simulink model "sf_tlevery"  (Simulink 6.0)
settings: Solver=ode45  StartTime=0.0  StopTime=100  RelTol=1e-3
settings Model: CovMetricSettings=dcmtr  Creator=The MathWorks Inc.  LastModifiedBy=batserve  ExtModeAutoUpdateStatusClock=off
settings OptimizationCC: BooleanDataType=off
settings DebuggingCC: CheckExecutionContextPreStartOutputMsg=on  CheckExecutionContextRuntimeOutputMsg=on  SolverPrmCheckMsg=none
settings HardwareCC: TargetUnknown=on

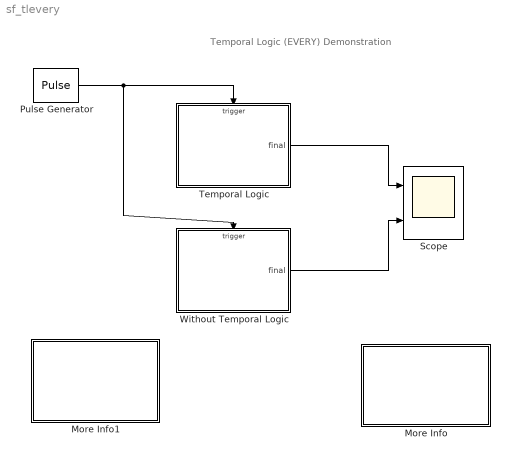
== system sf_tlevery ==
  note: Temporal Logic (EVERY) Demonstration
  More Info : Subsystem  PropExecContextAcrossSSBoundary=on
      mask Display: disp('Double click\nhere for\ninformation on\nthis demonstration')
  More Info1 : Subsystem  PropExecContextAcrossSSBoundary=on
      settings: OpenFcn=simcad(bdroot);
      mask Display: disp('Double click\nhere for\nSimulink\Stateflow\n Help')
  Pulse Generator : DiscretePulseGenerator  PulseType=Time based  Period=1  PulseWidth=.5
  Scope : Scope  NumInputPorts=2
      settings: TimeRange=100  YMin=-5~-5  YMax=40~40
  Temporal Logic : Stateflow chart  TreatAsAtomicUnit=on  PropExecContextAcrossSSBoundary=on
  Without Temporal Logic : Stateflow chart  TreatAsAtomicUnit=on  PropExecContextAcrossSSBoundary=on
  wires:
  Pulse Generator/1 -> Temporal Logic/Trigger, Without Temporal Logic/Trigger
  Temporal Logic/1(final) -> Scope/1
  Without Temporal Logic/1(final) -> Scope/2

== system sf_tlevery/More Info ==
  note: Temporal Logic using the EVERY function
  note: This demonstration illustrates the advantage of using the EVERY function to call a graphical function when
      | certain events occur. Notice how complicated it becomes when you try to accomplish the same behavior
      | without the use of temporal logic functions.
      |
      | In the Temporal Logic chart, we specify that every 5 secs (events), we will add one to the local variable
      | 'count'. We then say that every 10 secs, we will call the graphical function, double_counter, which is a function
      | that doubles its input, and give it the value of 'count', Notice that only one state and one graphical function
      | block are needed to accomplish this task when using temporal logic.
      |
      | In the Without Temporal Logic chart, we create the same behavior as the Temporal Logic chart. In order to
      | accomplish this, we need to use 4 state blocks and one graphical function block. Also, it becomes much more
      | difficult to follow the transitions and events that take place in the model. Again, the graphical function,
      | double_counter is called using 'count' as the input.

== system sf_tlevery/More Info1 ==

== stateflow chart Without Temporal Logic ==
  state Counter [parallel]
    state One
      count=1;
      One -> One : {count++;}
  state State [parallel]
    state A
    A -> (junction 12) : [count==5]{first_counter++;}
    (junction 12) -> A : {count=0;}
  state output = double_counter(input) [function]
    (default) -> (junction 13) : {output=2*input;}
  state State_two [parallel]
    state B
    B -> (junction 14) : [n==10]{final=double_counter(first_counter);}
    (junction 14) -> B : {n=0;}
  state Counter_two [parallel]
    state Two
      n=1;
      Two -> Two : {n++;}
  (default) -> A : {first_counter=0;}
  data: input function_input double; output function_output double; count local double; final output double; first_counter local double; n local double; m local double
  events: secs input RISING_EDGE_EVENT

== stateflow chart Temporal Logic ==
  state output = double_counter(input) [function]
    (default) -> (junction 35) : {output=2*input;}
  state Active
    on every(5,secs): count++;
    on every(10,secs):final=double_counter(count);
  (default) -> Active : {count=0;}
  data: input function_input double; output function_output double; count local double; final output double
  events: secs input RISING_EDGE_EVENT
